simulink model "power_aircraft_distribution_mexido"  (R2016a)
settings: Solver=VariableStepAuto  StartTime=0.0  StopTime=0.08  RelTol=1e-3
undefined symbols (not defined in the file or in its folder): D1, Delta, sigbuilder_block
libraries: powerlib x16, sps_avr x1, powerlib_meascontrol x1
settings Model: Creator=Joao  LastModifiedBy=Joao

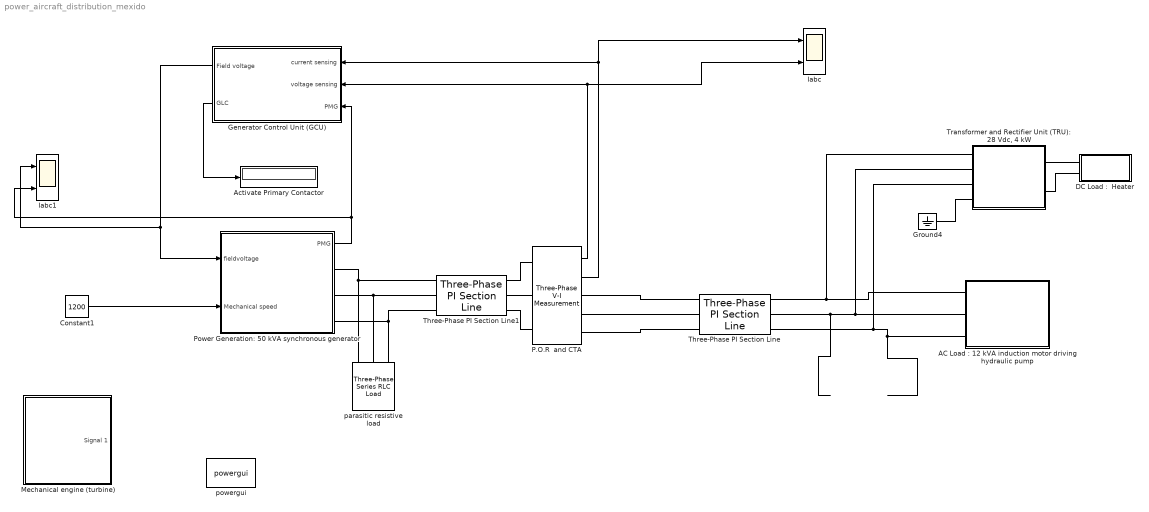
== system power_aircraft_distribution_mexido ==
  "AC Load : 12 kVA induction motor driving hydraulic pump" : Subsystem
      mask Display: image(imread('power_aircraft_distribution_EnginePump.jpg','jpg'))
  Activate Primary Contactor : Display
      settings: SampleTime=1e-2
  Constant1 : Constant  Value=1200
  "DC Load :  Heater" : Subsystem
      mask Display: image(imread('power_aircraft_distribution_heater.jpg','jpg'))
  Generator Control Unit (GCU) : Subsystem
      mask Display: image(imread('power_aircraft_distribution_GCU.jpg','jpg'))
  Ground4 : powerlib/Elements/Ground  LConnTagsString=a
  Iabc : Scope  NumInputPorts=2
  Iabc1 : Scope  NumInputPorts=2
  Mechanical engine (turbine) : Subsystem  Tag=STV Subsys  LoadFcn=sigbuilder_block('load');  StartFcn=sigbuilder_block('start');  StopFcn=sigbuilder_block('stop');  ClipboardFcn=sigbuilder_block('clipboard');  mask(Sigbuilder block){}
      mask help: Sigbuilder GUI
      mask init:
      | if ~strcmp(get_param(bdroot(gcbh),'SimulationStatus'),'stopped') tuvar = sigbuilder_block('maskInit'); end
      settings: CopyFcn=sigbuilder_block('copy');  DeleteFcn=sigbuilder_block('delete');  ModelCloseFcn=sigbuilder_block('modelClose');  PreSaveFcn=sigbuilder_block('preSave');  PauseFcn=sigbuilder_block('pause')  ContinueFcn=sigbuilder_block('continue')  NameChangeFcn=sigbuilder_block('namechange');  OpenFcn=sigbuilder_block('open',[5.4 5.4 1141.2 580.8 ]);  CloseFcn=sigbuilder_block('close');
      mask Display: image(imread('power_aircraft_distribution_turbine.jpg','jpg'))
  P.O.R  and CTA : powerlib/Measurements/Three-Phase V-I Measurement  VoltageMeasurement=phase-to-phase  SetLabelV=off  LabelV=Vabc  Vpu=off  VpuLL=off  CurrentMeasurement=yes  SetLabelI=off  LabelI=Iabc  Ipu=off  Pbase=100e6  Vbase=500e3  OutputType=Complex  PhasorSimulation=off  PSBequivalent=0
  Power Generation: 50 kVA synchronous generator : Subsystem
      mask Display: image(imread('power_aircraft_distribution_APU_Generator.jpg','jpg'))
  Three-Phase PI Section Line : powerlib/Elements/Three-Phase PI Section Line  LConnTagsString=a|b|c  RConnTagsString=A|B|C  Frequency=400  Resistances=[ 0.01273 0.3864]  Inductances="[ 0.9337e-3  4.1264e-3]"  Capacitances=[12.74e-9 7.751e-9]  Length=0.010
  Three-Phase PI Section Line1 : powerlib/Elements/Three-Phase PI Section Line  LConnTagsString=a|b|c  RConnTagsString=A|B|C  Frequency=400  Resistances=[ 0.01273 0.3864]  Inductances="[ 0.9337e-3  4.1264e-3]"  Capacitances=[12.74e-9 7.751e-9]  Length=0.010
  "Transformer and Rectifier Unit (TRU): 28 Vdc, 4 kW" : Subsystem
      mask Display: image(imread('power_aircraft_distribution_TRU.jpg','jpg'))
  parasitic resistive load : powerlib/Elements/Three-Phase Series RLC Load  LConnTagsString=A|B|C  Configuration=Y (grounded)  NominalVoltage=200  Vabc=[1e3 1e3 1e3]  Vabcp=[1e3 1e3 1e3]  NominalFrequency=400  UnbalancedPower=off  ActivePower=5000  InductivePower=0  CapacitivePower=0  Pabc=[10e3 9e3 11e3]  QLabc=[100 90 110]  QCabc=[100 90 110]  Pabcp=[10e3 9e3 11e3]  QLabcp=[100 90 110]  QCabcp=[100 90 110]  Measurements=None  LoadType=constant Z
  powergui : powerlib/powergui  Priority=1  SimulationMode=Discrete  SolverType=Tustin/Backward Euler (TBE)  SampleTime=1e-6  frequency=60  SPID=off  DisableSnubberDevices=off  DisableRonSwitches=off  DisableVfSwitches=off  SwTol=0  DisplayEquations=off  Interpol=off  ExternalGateDelay=off  methode=off  Ts=10  FunctionMessages=off  echomessages=off  HookPort=off  EnableUseOfTLC=off  x0status=blocks  frequencyindice=400  Pbase=100e6  ErrMax=1e-4  Iterations=50  UnitsV=kV  UnitsW=MW  buscounter=0  RestoreLinks=warning  ResistiveCurrentMeasurement=off  Frange=[0:2:500]  Ylog=off  Xlog=on  ShowGrid=off  save=off  variable=ZData  structure=0  ZoomFFT=off  StartTime=0.0  cycles=1  DisplayStyle=1  fundamental=60  FreqAxis=off  MaxFrequency=1000  frequencyindicesteady=1  RmsSteady=1  display=off
  wires:
  Power Generation: 50 kVA synchronous generator/1(PMG) -> Generator Control Unit (GCU)/3(PMG), Iabc1/2
  P.O.R  and CTA/1 -> Generator Control Unit (GCU)/2(voltage sensing), Iabc/2
  P.O.R  and CTA/2 -> Iabc/1, Generator Control Unit (GCU)/1(current sensing)
  Generator Control Unit (GCU)/2(GLC) -> Activate Primary Contactor/1
  Constant1/1 -> Power Generation: 50 kVA synchronous generator/2(Mechanical speed)
  Generator Control Unit (GCU)/1(Field voltage) -> Iabc1/1, Power Generation: 50 kVA synchronous generator/1(fieldvoltage)
  connections:
  Power Generation: 50 kVA synchronous generator/RConn1 -- Three-Phase PI Section Line1/LConn1 -- parasitic resistive load/LConn1
  Three-Phase PI Section Line/LConn2 -- P.O.R  and CTA/RConn2
  Three-Phase PI Section Line/LConn1 -- P.O.R  and CTA/RConn1
  Three-Phase PI Section Line/LConn3 -- P.O.R  and CTA/RConn3
  Three-Phase PI Section Line/RConn1 -- "Transformer and Rectifier Unit (TRU): 28 Vdc, 4 kW"/LConn1 -- "AC Load : 12 kVA induction motor driving hydraulic pump"/LConn1
  Three-Phase PI Section Line/RConn2 -- "Transformer and Rectifier Unit (TRU): 28 Vdc, 4 kW"/LConn2 -- "AC Load : 12 kVA induction motor driving hydraulic pump"/LConn2
  Three-Phase PI Section Line/RConn3 -- "Transformer and Rectifier Unit (TRU): 28 Vdc, 4 kW"/LConn3 -- "AC Load : 12 kVA induction motor driving hydraulic pump"/LConn3
  Power Generation: 50 kVA synchronous generator/RConn3 -- parasitic resistive load/LConn3 -- Three-Phase PI Section Line1/LConn3
  Power Generation: 50 kVA synchronous generator/RConn2 -- Three-Phase PI Section Line1/LConn2 -- parasitic resistive load/LConn2
  Three-Phase PI Section Line1/RConn1 -- P.O.R  and CTA/LConn1
  Three-Phase PI Section Line1/RConn2 -- P.O.R  and CTA/LConn2
  Three-Phase PI Section Line1/RConn3 -- P.O.R  and CTA/LConn3
  "Transformer and Rectifier Unit (TRU): 28 Vdc, 4 kW"/LConn4 -- Ground4/LConn1
  "DC Load :  Heater"/LConn1 -- "Transformer and Rectifier Unit (TRU): 28 Vdc, 4 kW"/RConn1
  "DC Load :  Heater"/LConn2 -- "Transformer and Rectifier Unit (TRU): 28 Vdc, 4 kW"/RConn2

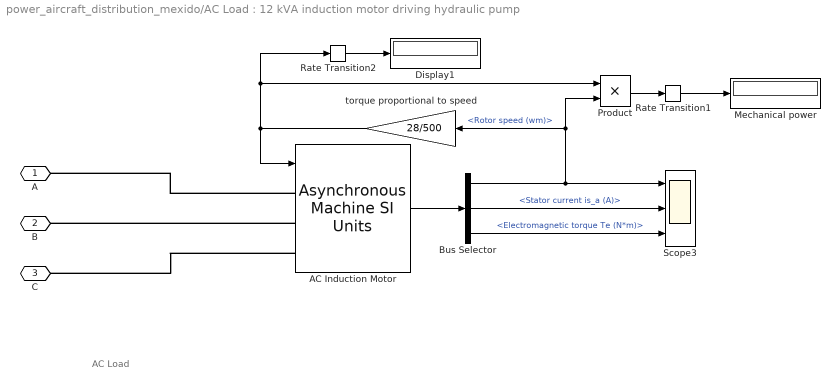
== system power_aircraft_distribution_mexido/AC Load : 12 kVA induction motor driving hydraulic pump ==
  note: AC Load
  AC Induction Motor : powerlib/Machines/Asynchronous Machine SI Units  RotorType=Squirrel-cage  PresetModel=No  MechanicalLoad=Torque Tm  ShowDetailedParameters=on  ReferenceFrame=Rotor  Units=SI  MeasurementBus=off  NominalParameters=[12e3 200 400]  Stator=[0.2761 0.002191/10]  Rotor=[0.16 0.002191/10]  Cage1=[ 0.022 0.226/377]  Cage2=[ 0.022 0.226/377]  Lm=0.07614  Mechanical=[0.01 0 8]  PolePairs=8  InitialConditions=[1,0 0,0,0 0,0,0]  SimulateSaturation=off  Saturation=[14.03593122, 27.81365428, 53.79336849, 72.68890987, 97.98006896, 148.6815601, 215.7428561, 302.9841135, 428.7778367 ; 230, 322, 414, 460, 506, 552, 598, 644, 690]  LoadFlowParameters=0  TsPowergui=0  TsBlock=-1  IterativeModel=Trapezoidal non iterative  IterativeDiscreteModel=Trapezoidal non iterative  Pmec=0
  Bus Selector : BusSelector  OutputSignals=Mechanical.Rotor speed (wm),Stator measurements.Stator current is_a (A),Mechanical.Electromagnetic torque Te (N*m)
  Display1 : Display
      settings: SampleTime=1e-2
  Mechanical power : Display
      settings: SampleTime=1e-2
  Product : Product  RndMeth=Zero
  Rate Transition1 : RateTransition  OutPortSampleTimeOpt=Inherit  OutPortSampleTime=Ts
  Rate Transition2 : RateTransition  OutPortSampleTimeOpt=Inherit  OutPortSampleTime=Ts
  Scope3 : Scope  NumInputPorts=3
  torque proportional to speed : Gain  Gain=28/500
  A : PMIOPort  Port=1  Side=Left
  B : PMIOPort  Port=2  Side=Left
  C : PMIOPort  Port=3  Side=Left
  wires:
  AC Induction Motor/1 -> Bus Selector/1
  Bus Selector/1 -> Scope3/1, torque proportional to speed/1, Product/2  "<Rotor speed (wm)>"
  torque proportional to speed/1 -> AC Induction Motor/1, Product/1, Rate Transition2/1
  Product/1 -> Rate Transition1/1
  Bus Selector/2 -> Scope3/2  "<Stator current is_a (A)>"
  Bus Selector/3 -> Scope3/3  "<Electromagnetic torque Te (N*m)>"
  Rate Transition1/1 -> Mechanical power/1
  Rate Transition2/1 -> Display1/1
  connections:
  AC Induction Motor/LConn2 -- B/RConn1
  AC Induction Motor/LConn1 -- A/RConn1
  AC Induction Motor/LConn3 -- C/RConn1

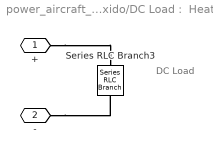
== system power_aircraft_distribution_mexido/DC Load :  Heater ==
  note: DC Load
  Series RLC Branch3 : powerlib/Elements/Series RLC Branch  LConnTagsString=__new0  RConnTagsString=__new0  BranchType=R  Resistance=1  Inductance=[]  SetiL0=off  InitialCurrent=0  Capacitance=[]  Setx0=off  InitialVoltage=0  Measurements=Branch voltage and current
  + : PMIOPort  Port=1  Side=Left
  - : PMIOPort  Port=2  Side=Left
  connections:
  -/RConn1 -- Series RLC Branch3/RConn1
  +/RConn1 -- Series RLC Branch3/LConn1

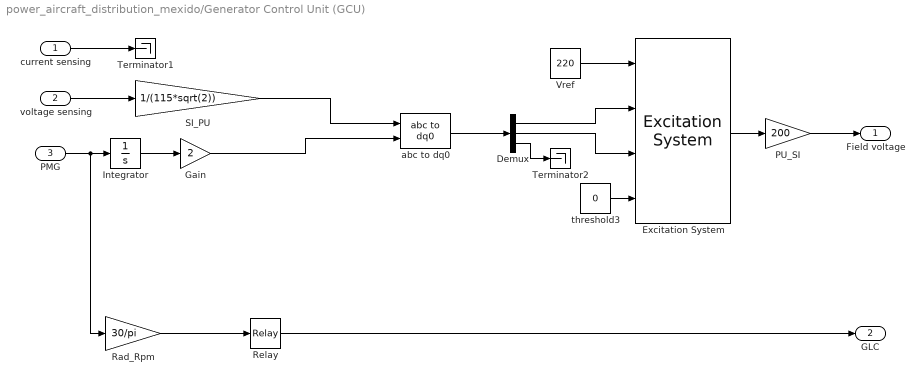
== system power_aircraft_distribution_mexido/Generator Control Unit (GCU) ==
  current sensing : Inport
  voltage sensing : Inport  Port=2
  PMG : Inport  Port=3
  Demux : Demux  Outputs=3
  Excitation System : sps_avr/Excitation System  tr=20e-3  reg=[ 300, 0.001 ]  exc=[ 1, 0 ]  tgr=[ 0, 0 ]  damp=[ 0.001, 0.1 ]  sat=[ 0, 0 ]  lim=[ -2, 2, 0 ]  v0=[1 0]
  Gain : Gain  Gain=2
  Integrator : Integrator
  PU_SI : Gain  Gain=200
  Rad_Rpm : Gain  Gain=30/pi
  Relay : Relay  OnSwitchValue=9000  OffSwitchValue=8900
  SI_PU : Gain  Gain=1/(115*sqrt(2))
  Terminator1 : Terminator
  Terminator2 : Terminator
  Vref : Constant  Value=220
  abc to dq0 : powerlib_meascontrol/Transformations/abc to dq0  Alignment=90 degrees behind phase A axis
  threshold3 : Constant  Value=0
  Field voltage : Outport
  GLC : Outport  Port=2
  wires:
  Relay/1 -> GLC/1
  Demux/3 -> Terminator2/1
  current sensing/1 -> Terminator1/1
  threshold3/1 -> Excitation System/4
  Vref/1 -> Excitation System/1
  Rad_Rpm/1 -> Relay/1
  PU_SI/1 -> Field voltage/1
  Excitation System/1 -> PU_SI/1
  SI_PU/1 -> abc to dq0/1
  Demux/2 -> Excitation System/3
  Demux/1 -> Excitation System/2
  abc to dq0/1 -> Demux/1
  Integrator/1 -> Gain/1
  voltage sensing/1 -> SI_PU/1
  PMG/1 -> Rad_Rpm/1, Integrator/1
  Gain/1 -> abc to dq0/2

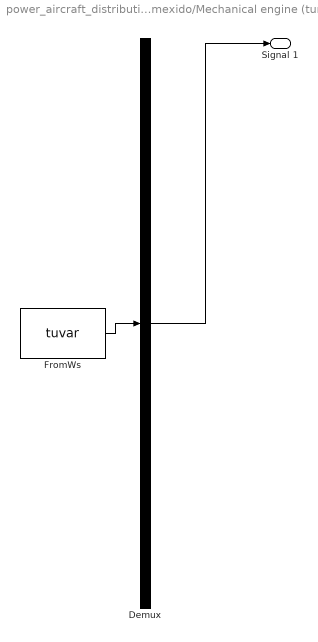
== system power_aircraft_distribution_mexido/Mechanical engine (turbine) ==
  Demux : Demux  Tag=STV Demux  Outputs=1
  FromWs : FromWorkspace  Tag=STV FromWs  VariableName=tuvar  SampleTime=0
      SigBuilderData=|
      | common.afterFinalStr = 'Extrapolate'
      | common.sampleTime = 0
      | dataSet.timeRange = [0 10]
      | dataSet.name = 'Group 1'
      | sbobj.Groups.Name = 'Group 1'
      | sbobj.Groups.Signals.Name = 'Signal 1'
      | sbobj.Groups.Signals.XData = [0 0.4 0.5 1 2 3 4.5 6 6 10]
      | sbobj.Groups.Signals.YData = [0 12000 12000 12000 12000 10000 18000 1 0 0]
  Signal 1 : Outport  Tag=STV Outport
  wires:
  FromWs/1 -> Demux/1
  Demux/1 -> Signal 1/1

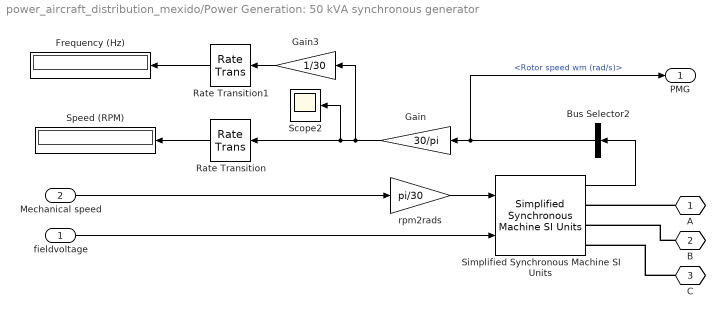
== system power_aircraft_distribution_mexido/Power Generation: 50 kVA synchronous generator ==
  fieldvoltage : Inport
  Mechanical speed : Inport  Port=2
  Bus Selector2 : BusSelector  OutputSignals=Rotor speed wm (rad/s)
  Frequency (Hz) : Display
      settings: SampleTime=1e-2
  Gain : Gain  Gain=30/pi
  Gain3 : Gain  Gain=1/30
  Rate Transition : RateTransition  OutPortSampleTimeOpt=Inherit  OutPortSampleTime=Ts
  Rate Transition1 : RateTransition  OutPortSampleTimeOpt=Inherit  OutPortSampleTime=Ts
  Scope2 : Scope
  Simplified Synchronous Machine SI Units : powerlib/Machines/Simplified Synchronous Machine SI Units  ConnectionType=3-wire Y  MechanicalLoad=Speed w  MeasurementBus=off  NominalParameters=[50e3 200 400]  Mechanical=[0.02 0 2]  InternalRL="[0.0204  0.08104e-3]"  InitialConditions=[-99,0 0,0,0 0,0,0]  Units=1  LoadFlowParameters=[1 0 0 0 0]  TsPowergui=0  TsBlock=Ts  BusType=PV  Pref=0  Qref=0  Qmin=-inf  Qmax=+inf  PLF=0  QLF=0
  Speed (RPM) : Display
      settings: SampleTime=1e-2
  rpm2rads : Gain  Gain=pi/30
  A : PMIOPort  Tag=PMCPort  Port=1  Side=Right
  B : PMIOPort  Tag=PMCPort  Port=2  Side=Right
  C : PMIOPort  Tag=PMCPort  Port=3  Side=Right
  PMG : Outport
  wires:
  Simplified Synchronous Machine SI Units/1 -> Bus Selector2/1
  fieldvoltage/1 -> Simplified Synchronous Machine SI Units/2
  Bus Selector2/1 -> Gain/1, PMG/1  "<Rotor speed wm (rad/s)>"
  Gain/1 -> Gain3/1, Scope2/1, Rate Transition/1
  Gain3/1 -> Rate Transition1/1
  Mechanical speed/1 -> rpm2rads/1
  rpm2rads/1 -> Simplified Synchronous Machine SI Units/1
  Rate Transition/1 -> Speed (RPM)/1
  Rate Transition1/1 -> Frequency (Hz)/1
  connections:
  A/RConn1 -- Simplified Synchronous Machine SI Units/RConn1
  B/RConn1 -- Simplified Synchronous Machine SI Units/RConn2
  C/RConn1 -- Simplified Synchronous Machine SI Units/RConn3

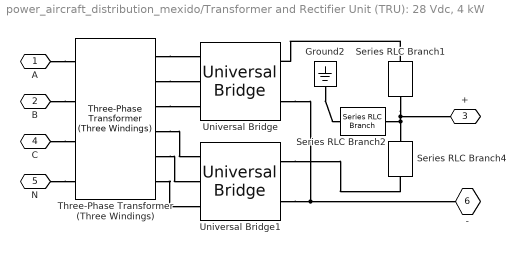
== system power_aircraft_distribution_mexido/Transformer and Rectifier Unit (TRU): 28 Vdc, 4 kW ==
  Ground2 : powerlib/Elements/Ground  LConnTagsString=a
  Series RLC Branch1 : powerlib/Elements/Series RLC Branch  LConnTagsString=__new0  RConnTagsString=__new0  BranchType=L  Resistance=[]  Inductance=2e-3  SetiL0=on  InitialCurrent=0  Capacitance=[]  Setx0=off  InitialVoltage=0  Measurements=Branch voltage and current
  Series RLC Branch2 : powerlib/Elements/Series RLC Branch  LConnTagsString=__new0  RConnTagsString=__new0  BranchType=C  Resistance=[]  Inductance=[]  SetiL0=off  InitialCurrent=0  Capacitance=1e-6  Setx0=off  InitialVoltage=0  Measurements=None
  Series RLC Branch4 : powerlib/Elements/Series RLC Branch  LConnTagsString=__new0  RConnTagsString=__new0  BranchType=L  Resistance=[]  Inductance=2e-3  SetiL0=off  InitialCurrent=0  Capacitance=[]  Setx0=off  InitialVoltage=0  Measurements=Branch voltage and current
  Three-Phase Transformer (Three Windings) : powerlib/Elements/Three-Phase Transformer (Three Windings)  Winding1Connection=Yn  Winding2Connection=Delta (D1)  Winding3Connection=Delta (D1)  CoreType=Three single-phase transformers  SetSaturation=off  Hysteresis=off  DataFile='hysteresis'  SetInitialFlux=off  Measurements=None  UNITS=pu  NominalPower=[ 4200 , 600 ]  Winding1=[ 200 , 0.0002 , 0 ]  Winding2=[ 22 , 0.0002 , 0 ]  Winding3=[ 22 , 0.0002 , 0]  Rm=500  Lm=500*10  L0=0.5  Saturation=[ 0,0 ; 0.0024,1.2 ; 1.0,1.52 ]  InitialFluxes=[0.8 -0.8 0.7]  MoreParameters=off  BreakLoop=off  DataType=off  TransfoNumber=0
  Universal Bridge : powerlib/Power Electronics/Universal Bridge  Arms=3  SnubberResistance=1e3  SnubberCapacitance=1e-6  Device=Diodes  Ron=1e-3  Lon=0  ForwardVoltages="[  0  0  ]"  ForwardVoltage=0.8  GTOparameters=[ 10e-6 , 20e-6 ]  IGBTparameters=[ 1e-6 , 2e-6 ]  Measurements=None  Measurements_2=None  converterType=Rectifier
  Universal Bridge1 : powerlib/Power Electronics/Universal Bridge  Arms=3  SnubberResistance=1e3  SnubberCapacitance=1e-6  Device=Diodes  Ron=1e-3  Lon=0  ForwardVoltages="[  0  0  ]"  ForwardVoltage=0.8  GTOparameters=[ 10e-6 , 20e-6 ]  IGBTparameters=[ 1e-6 , 2e-6 ]  Measurements=None  Measurements_2=None  converterType=Rectifier
  A : PMIOPort  Port=1  Side=Left
  B : PMIOPort  Port=2  Side=Left
  + : PMIOPort  Port=3  Side=Right
  C : PMIOPort  Port=4  Side=Left
  N : PMIOPort  Port=5  Side=Left
  - : PMIOPort  Port=6  Side=Right
  connections:
  Ground2/LConn1 -- Series RLC Branch2/RConn1
  Universal Bridge/RConn2 -- Universal Bridge1/RConn2 -- -/RConn1
  Three-Phase Transformer (Three Windings)/RConn1 -- Universal Bridge/LConn1
  Three-Phase Transformer (Three Windings)/RConn2 -- Universal Bridge/LConn2
  Three-Phase Transformer (Three Windings)/RConn3 -- Universal Bridge/LConn3
  A/RConn1 -- Three-Phase Transformer (Three Windings)/LConn1
  B/RConn1 -- Three-Phase Transformer (Three Windings)/LConn2
  C/RConn1 -- Three-Phase Transformer (Three Windings)/LConn3
  N/RConn1 -- Three-Phase Transformer (Three Windings)/LConn4
  Series RLC Branch1/LConn1 -- Universal Bridge/RConn1
  Series RLC Branch2/LConn1 -- Series RLC Branch1/RConn1 -- +/RConn1 -- Series RLC Branch4/LConn1
  Three-Phase Transformer (Three Windings)/RConn4 -- Universal Bridge1/LConn1
  Three-Phase Transformer (Three Windings)/RConn5 -- Universal Bridge1/LConn2
  Three-Phase Transformer (Three Windings)/RConn6 -- Universal Bridge1/LConn3
  Universal Bridge1/RConn1 -- Series RLC Branch4/RConn1
